simulink model "the3TankSim"  (R2024a)
settings: Solver=FixedStepAuto  StartTime=0.0  StopTime=80000  FixedStep=1  RelTol=1e-3
values from neighbouring files (symbols this model uses):
  A = 1    [init3TankSim.m]    (also in tankParameters.mat)
  h1init = 10    [init3TankSim.m]    (also in tankParameters.mat = 0)
  h2init = 10    [init3TankSim.m]    (also in tankParameters.mat = 0)
  h3init = 10    [init3TankSim.m]    (also in tankParameters.mat = 0)
  Ktb1to2 = 0.0334    [init3TankSim.m]    (also in tankParameters.mat)
  Ktb2to3 = 0.0334    [init3TankSim.m]    (also in tankParameters.mat)
  Kv1out = 0.02727    [init3TankSim.m]    (also in tankParameters.mat)
  Kv1to2 = 0.075    [init3TankSim.m]    (also in tankParameters.mat)
  Kv2out = 0.0045    [init3TankSim.m]    (also in tankParameters.mat)
  Kv2to3 = 0.075    [init3TankSim.m]    (also in tankParameters.mat)
  Kv3out = 0.02727    [init3TankSim.m]    (also in tankParameters.mat)
  Tube1to2onoff = 1    [init3TankSim.m]    (also in tankParameters.mat)
  Tube2to3onoff = 1    [init3TankSim.m]    (also in tankParameters.mat)
settings Model: Creator=Kleinmann  LastModifiedBy=elfridaanindya
settings SolverCC: AlgebraicLoopSolver=TrustRegion
settings DebuggingCC: UnconnectedInputMsg=warning  UnconnectedOutputMsg=warning  UnconnectedLineMsg=warning
settings ModelReferenceCC: EnableRefExpFcnMdlSchedulingChecks=on
settings RTWCC: GPUComputeCapability=3.5  DLArmComputeVersion=19.05

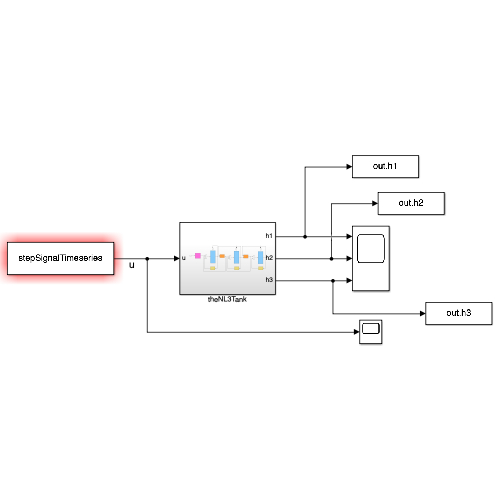
[thumbnail: Simulink's stored preview of the top-level diagram]
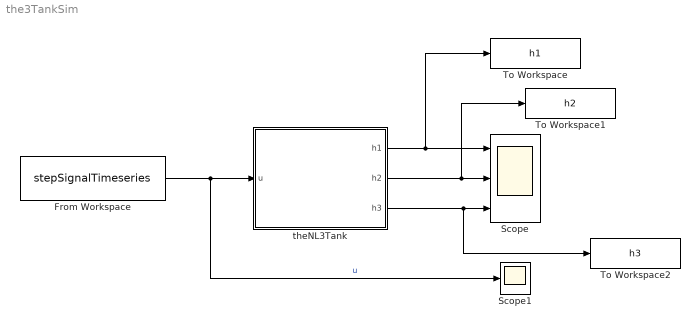
== system the3TankSim ==
  From Workspace : FromWorkspace  VariableName=stepSignalTimeseries  SampleTime=1  OutputAfterFinalValue=Setting to zero
  Scope : Scope  NumInputPorts=3
  Scope1 : Scope
  To Workspace : ToWorkspace  VariableName=h1  SampleTime=-1
  To Workspace1 : ToWorkspace  VariableName=h2  SampleTime=-1
  To Workspace2 : ToWorkspace  VariableName=h3  SampleTime=-1
  theNL3Tank : Subsystem
  wires:
  theNL3Tank/1(h1) -> To Workspace/1, Scope/1
  theNL3Tank/2(h2) -> To Workspace1/1, Scope/2
  theNL3Tank/3(h3) -> To Workspace2/1, Scope/3
  From Workspace/1 -> Scope1/1, theNL3Tank/1(u)  "u"

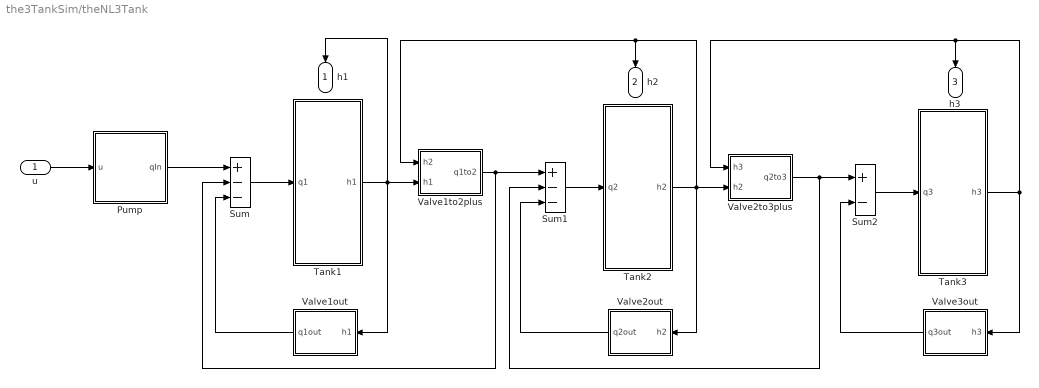
== system the3TankSim/theNL3Tank ==
  u : Inport
  Pump : Subsystem
  Sum : Sum  Inputs=+--
  Sum1 : Sum  Inputs=+--
  Sum2 : Sum  Inputs=+-
  Tank1 : Subsystem
  Tank2 : Subsystem
  Tank3 : Subsystem
  Valve1out : Subsystem
  Valve1to2plus : Subsystem
  Valve2out : Subsystem
  Valve2to3plus : Subsystem
  Valve3out : Subsystem
  h1 : Outport
  h2 : Outport  Port=2
  h3 : Outport  Port=3
  wires:
  u/1 -> Pump/1(u)
  Tank1/1(h1) -> h1/1, Valve1out/1(h1), Valve1to2plus/2(h1)
  Tank2/1(h2) -> Valve2to3plus/2(h2), h2/1, Valve1to2plus/1(h2), Valve2out/1(h2)
  Valve1to2plus/1(q1to2) -> Sum1/1, Sum/2
  Valve2out/1(q2out) -> Sum1/3
  Valve1out/1(q1out) -> Sum/3
  Valve3out/1(q3out) -> Sum2/2
  Tank3/1(h3) -> Valve2to3plus/1(h3), h3/1, Valve3out/1(h3)
  Valve2to3plus/1(q2to3) -> Sum2/1, Sum1/2
  Pump/1(qIn) -> Sum/1
  Sum1/1 -> Tank2/1(q2)
  Sum2/1 -> Tank3/1(q3)
  Sum/1 -> Tank1/1(q1)

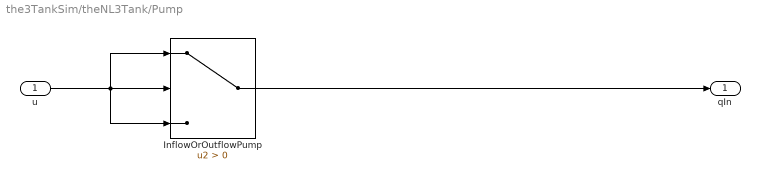
== system the3TankSim/theNL3Tank/Pump ==
  u : Inport
  InflowOrOutflowPump : Switch  Criteria=u2 > Threshold  SaturateOnIntegerOverflow=off  InputSameDT=off
  qIn : Outport
  wires:
  u/1 -> InflowOrOutflowPump/1, InflowOrOutflowPump/3, InflowOrOutflowPump/2
  InflowOrOutflowPump/1 -> qIn/1

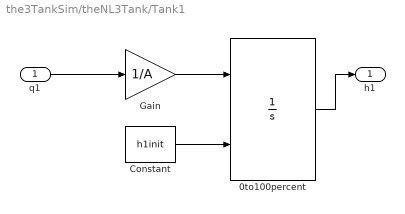
== system the3TankSim/theNL3Tank/Tank1 ==
  q1 : Inport
  0to100percent : Integrator  InitialConditionSource=external  LimitOutput=on  UpperSaturationLimit=100  LowerSaturationLimit=0
  Constant : Constant  Value=h1init
  Gain : Gain  Gain=1/A
  h1 : Outport
  wires:
  0to100percent/1 -> h1/1
  Gain/1 -> 0to100percent/1
  Constant/1 -> 0to100percent/2
  q1/1 -> Gain/1

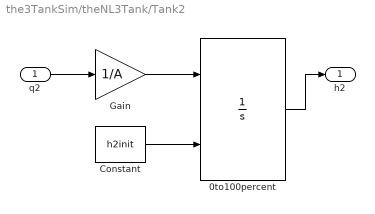
== system the3TankSim/theNL3Tank/Tank2 ==
  q2 : Inport
  0to100percent : Integrator  InitialConditionSource=external  LimitOutput=on  UpperSaturationLimit=100  LowerSaturationLimit=0
  Constant : Constant  Value=h2init
  Gain : Gain  Gain=1/A
  h2 : Outport
  wires:
  Constant/1 -> 0to100percent/2
  Gain/1 -> 0to100percent/1
  0to100percent/1 -> h2/1
  q2/1 -> Gain/1

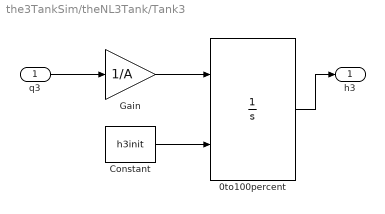
== system the3TankSim/theNL3Tank/Tank3 ==
  q3 : Inport
  0to100percent : Integrator  InitialConditionSource=external  LimitOutput=on  UpperSaturationLimit=100  LowerSaturationLimit=0
  Constant : Constant  Value=h3init
  Gain : Gain  Gain=1/A
  h3 : Outport
  wires:
  q3/1 -> Gain/1
  Constant/1 -> 0to100percent/2
  Gain/1 -> 0to100percent/1
  0to100percent/1 -> h3/1

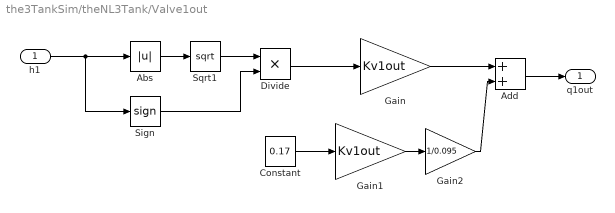
== system the3TankSim/theNL3Tank/Valve1out ==
  h1 : Inport
  Abs : Abs  SaturateOnIntegerOverflow=off
  Add : Sum
  Constant : Constant  Value=0.17
  Divide : Product
  Gain : Gain  Gain=Kv1out
  Gain1 : Gain  Gain=Kv1out
  Gain2 : Gain  Gain=1/0.095
  Sign : Signum
  Sqrt1 : Sqrt
  q1out : Outport
  wires:
  Sqrt1/1 -> Divide/1
  Sign/1 -> Divide/2
  h1/1 -> Sign/1, Abs/1
  Abs/1 -> Sqrt1/1
  Gain/1 -> Add/1
  Add/1 -> q1out/1
  Gain1/1 -> Gain2/1
  Gain2/1 -> Add/2
  Constant/1 -> Gain1/1
  Divide/1 -> Gain/1

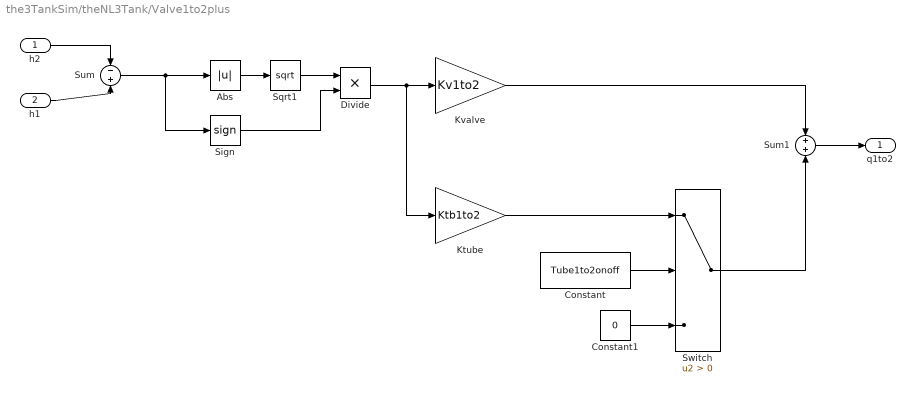
== system the3TankSim/theNL3Tank/Valve1to2plus ==
  h2 : Inport
  h1 : Inport  Port=2
  Abs : Abs  SaturateOnIntegerOverflow=off
  Constant : Constant  Value=Tube1to2onoff
  Constant1 : Constant  Value=0
  Divide : Product
  Ktube : Gain  Gain=Ktb1to2
  Kvalve : Gain  Gain=Kv1to2
  Sign : Signum
  Sqrt1 : Sqrt
  Sum : Sum  Inputs=-+
  Sum1 : Sum
  Switch : Switch  Criteria=u2 > Threshold  SaturateOnIntegerOverflow=off  InputSameDT=off
  q1to2 : Outport
  wires:
  h1/1 -> Sum/2
  h2/1 -> Sum/1
  Sum/1 -> Sign/1, Abs/1
  Kvalve/1 -> Sum1/1
  Sum1/1 -> q1to2/1
  Divide/1 -> Ktube/1, Kvalve/1
  Switch/1 -> Sum1/2
  Constant/1 -> Switch/2
  Ktube/1 -> Switch/1
  Constant1/1 -> Switch/3
  Abs/1 -> Sqrt1/1
  Sqrt1/1 -> Divide/1
  Sign/1 -> Divide/2

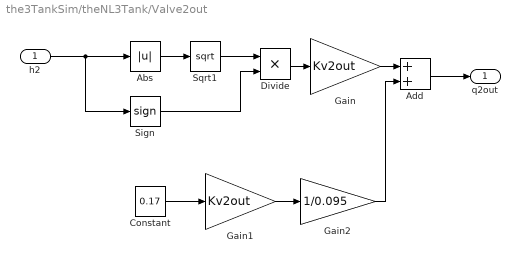
== system the3TankSim/theNL3Tank/Valve2out ==
  h2 : Inport
  Abs : Abs  SaturateOnIntegerOverflow=off
  Add : Sum
  Constant : Constant  Value=0.17
  Divide : Product
  Gain : Gain  Gain=Kv2out
  Gain1 : Gain  Gain=Kv2out
  Gain2 : Gain  Gain=1/0.095
  Sign : Signum
  Sqrt1 : Sqrt
  q2out : Outport
  wires:
  Divide/1 -> Gain/1
  Sqrt1/1 -> Divide/1
  Sign/1 -> Divide/2
  h2/1 -> Sign/1, Abs/1
  Abs/1 -> Sqrt1/1
  Gain2/1 -> Add/2
  Gain/1 -> Add/1
  Add/1 -> q2out/1
  Constant/1 -> Gain1/1
  Gain1/1 -> Gain2/1

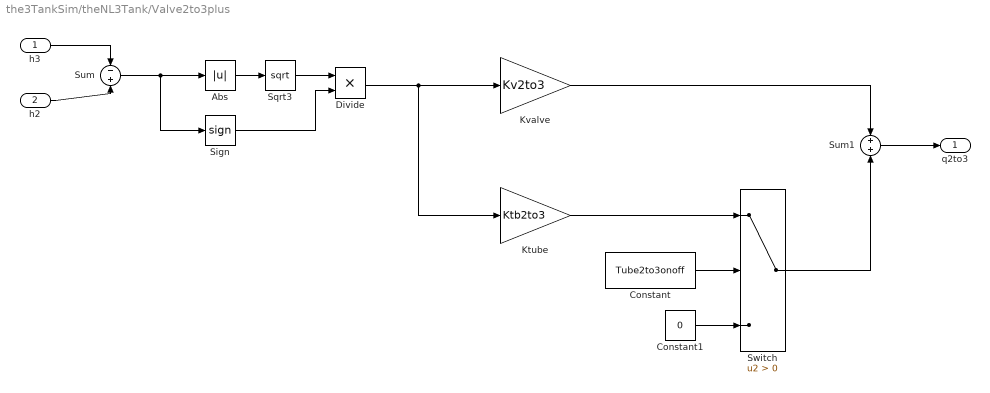
== system the3TankSim/theNL3Tank/Valve2to3plus ==
  h3 : Inport
  h2 : Inport  Port=2
  Abs : Abs  SaturateOnIntegerOverflow=off
  Constant : Constant  Value=Tube2to3onoff
  Constant1 : Constant  Value=0
  Divide : Product
  Ktube : Gain  Gain=Ktb2to3
  Kvalve : Gain  Gain=Kv2to3
  Sign : Signum
  Sqrt3 : Sqrt
  Sum : Sum  Inputs=-+
  Sum1 : Sum
  Switch : Switch  Criteria=u2 > Threshold  SaturateOnIntegerOverflow=off  InputSameDT=off
  q2to3 : Outport
  wires:
  Sum1/1 -> q2to3/1
  Kvalve/1 -> Sum1/1
  Ktube/1 -> Switch/1
  Constant1/1 -> Switch/3
  Divide/1 -> Ktube/1, Kvalve/1
  Switch/1 -> Sum1/2
  Constant/1 -> Switch/2
  h2/1 -> Sum/2
  h3/1 -> Sum/1
  Sqrt3/1 -> Divide/1
  Sign/1 -> Divide/2
  Sum/1 -> Sign/1, Abs/1
  Abs/1 -> Sqrt3/1

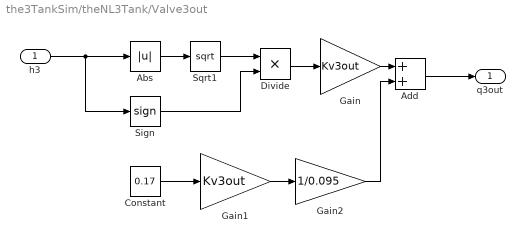
== system the3TankSim/theNL3Tank/Valve3out ==
  h3 : Inport
  Abs : Abs  SaturateOnIntegerOverflow=off
  Add : Sum
  Constant : Constant  Value=0.17
  Divide : Product
  Gain : Gain  Gain=Kv3out
  Gain1 : Gain  Gain=Kv3out
  Gain2 : Gain  Gain=1/0.095
  Sign : Signum
  Sqrt1 : Sqrt
  q3out : Outport
  wires:
  Sqrt1/1 -> Divide/1
  Sign/1 -> Divide/2
  h3/1 -> Sign/1, Abs/1
  Abs/1 -> Sqrt1/1
  Divide/1 -> Gain/1
  Gain/1 -> Add/1
  Gain2/1 -> Add/2
  Add/1 -> q3out/1
  Gain1/1 -> Gain2/1
  Constant/1 -> Gain1/1
